simulink model "lab3_4_4-1"  (R2021b)
settings: Solver=VariableStepAuto  StartTime=0.0  StopTime=10.0  RelTol=1e-3
libraries: nonlinear_cart x1
settings Model: Creator=adanm  LastModifiedBy=Juho
settings SolverCC: AlgebraicLoopSolver=TrustRegion
settings DataIOCC: ReturnWorkspaceOutputs=off
settings DebuggingCC: SFMachineParentedDataDiag=warning  ArithmeticOperatorsInVariantConditions=warning
settings SFSimCC: CustomCodeUndefinedFunction=UseInterfaceOnly

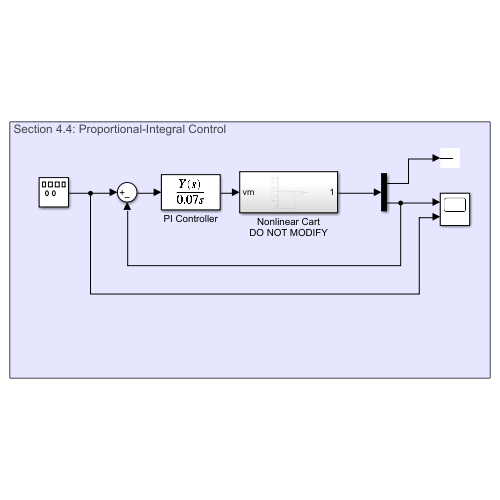
[thumbnail: Simulink's stored preview of the top-level diagram]
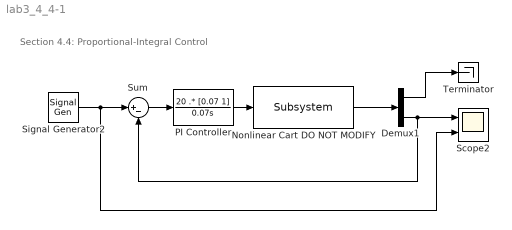
== system lab3_4_4-1 ==
  note: Section 4.4: Proportional-Integral Control
  Demux1 : Demux  Outputs=2
  Nonlinear Cart DO NOT MODIFY : nonlinear_cart/Subsystem  SystemSampleTime=-1  VariantActivationTime=update diagram  Latency=0  AutoFrameSizeCalculation=off
  PI Controller : TransferFcn  Numerator=20 .* [0.07 1]  Denominator=[0.07 0]
  Scope2 : Scope  NumInputPorts=2
  Signal Generator2 : SignalGenerator  WaveForm=square  Amplitude=0.2  Frequency=0.5
  Sum : Sum  Inputs=|+-
  Terminator : Terminator
  wires:
  Nonlinear Cart DO NOT MODIFY/1 -> Demux1/1
  Demux1/1 -> Terminator/1
  PI Controller/1 -> Nonlinear Cart DO NOT MODIFY/1
  Demux1/2 -> Sum/2, Scope2/1
  Signal Generator2/1 -> Scope2/2, Sum/1
  Sum/1 -> PI Controller/1
